simulink model "ls_fault_sw_4rt_10khz_bis"  (R2025a)
settings: Solver=VariableStepAuto  StartTime=0.0  StopTime=0.3  MaxStep=1/10e3  RelTol=1e-3
values from neighbouring files (symbols this model uses):
  Tsmpl = 1/(ovsmpl*fsw)    (= 5e-06)    [sim_ls_fault_init_4rt_10khz.m]
undefined symbols (not defined in the file or in its folder): plecs
settings Model: Creator=mem21  LastModifiedBy=mem21
settings DataIOCC: ReturnWorkspaceOutputs=off
settings OptimizationCC: DefaultParameterBehavior=Inlined  GainParamInheritBuiltInType=on  UseFloatMulNetSlope=on  InlineInvariantSignals=on  EfficientFloat2IntCast=on
settings DebuggingCC: SignalInfNanChecking=warning  AlgebraicLoopMsg=none
settings RTWCC: GenCodeOnly=on  BuildConfiguration=Faster Runs
settings GRTTargetCC: MatFileLogging=off  SupportNonFinite=off

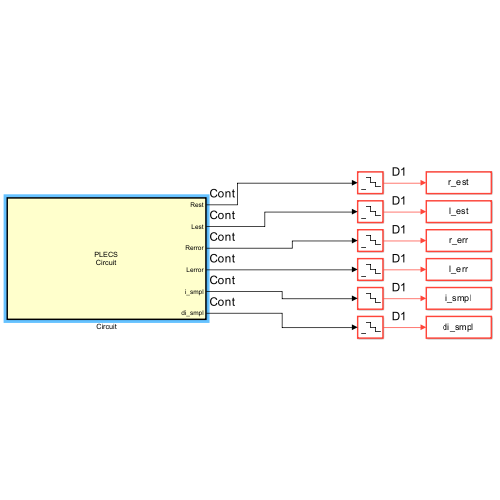
[thumbnail: Simulink's stored preview of the top-level diagram]
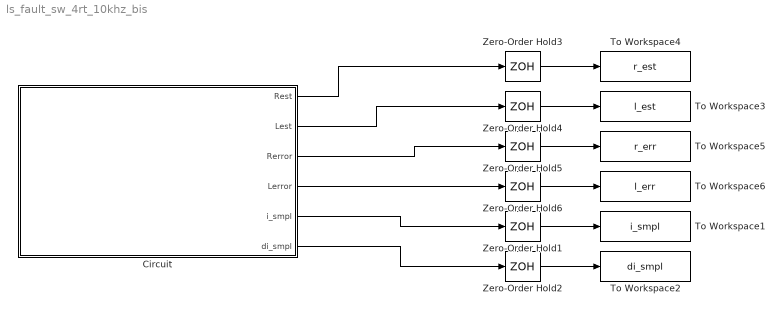
== system ls_fault_sw_4rt_10khz_bis ==
  Circuit : Subsystem  LoadFcn=plecs('sl', 200);  InitFcn=plecs('sl', 214);  StartFcn=plecs('sl', 208);  StopFcn=plecs('sl', 209);  mask(PlecsCircuit){PLECSData=<binary blob, 34132 chars, not shown>}
      mask prompts: PLECSData "PLECS Data (Do not delete or modify!)"
      mask init:
      | % PLACE CUSTOM INITIALIZATIONS ABOVE
      | % DO NOT REMOVE
      | plecs('sl', 215);
      | % DO NOT REMOVE
      settings: CopyFcn=plecs('sl', 203);  DeleteFcn=plecs('sl', 205);  UndoDeleteFcn=plecs('sl', 206);  PreSaveFcn=plecs('sl', 211);  PostSaveFcn=plecs('sl', 201);  NameChangeFcn=plecs('sl', 210);  DestroyFcn=plecs('sl', 207);  PreCopyFcn=plecs('sl', 216);  OpenFcn=plecs('sl', 202);  ErrorFcn=plerrorfcn
      mask Help: eval('plecs(''help'', ''qthelp:///creatingacircuit.html'')')
      mask Display: disp('PLECS\nCircuit')
  To Workspace1 : ToWorkspace  VariableName=i_smpl  SaveFormat=Structure With Time  SampleTime=-1
  To Workspace2 : ToWorkspace  VariableName=di_smpl  SaveFormat=Structure With Time  SampleTime=-1
  To Workspace3 : ToWorkspace  VariableName=l_est  SaveFormat=Structure With Time  SampleTime=-1
  To Workspace4 : ToWorkspace  VariableName=r_est  SaveFormat=Structure With Time  SampleTime=-1
  To Workspace5 : ToWorkspace  VariableName=r_err  SaveFormat=Structure With Time  SampleTime=-1
  To Workspace6 : ToWorkspace  VariableName=l_err  SaveFormat=Structure With Time  SampleTime=-1
  Zero-Order Hold{1..6} (6 alike) : ZeroOrderHold  SampleTime=Tsmpl
  wires:
  Zero-Order Hold4/1 -> To Workspace3/1
  Zero-Order Hold5/1 -> To Workspace5/1
  Zero-Order Hold3/1 -> To Workspace4/1
  Zero-Order Hold6/1 -> To Workspace6/1
  Circuit/1(Rest) -> Zero-Order Hold3/1
  Circuit/2(Lest) -> Zero-Order Hold4/1
  Circuit/3(Rerror) -> Zero-Order Hold5/1
  Circuit/4(Lerror) -> Zero-Order Hold6/1
  Zero-Order Hold1/1 -> To Workspace1/1
  Zero-Order Hold2/1 -> To Workspace2/1
  Circuit/5(i_smpl) -> Zero-Order Hold1/1
  Circuit/6(di_smpl) -> Zero-Order Hold2/1

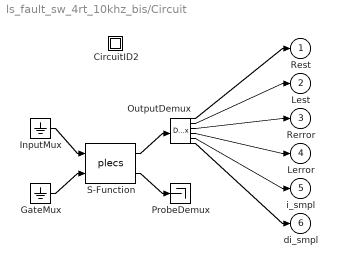
== system ls_fault_sw_4rt_10khz_bis/Circuit ==
  " CircuitID2 " : Subsystem
  " GateMux " : Ground
  " InputMux " : Ground
  " OutputDemux " : Demux  Outputs=[ 1 1 1 1 1 1 ]
  " ProbeDemux " : Terminator
  " S-Function " : S-Function  FunctionName=plecs  SFunctionDeploymentMode=off  EnableBusSupport=off
  Rest : Outport  PortDimensions=1
  Lest : Outport  Port=2  PortDimensions=1
  Rerror : Outport  Port=3  PortDimensions=1
  Lerror : Outport  Port=4  PortDimensions=1
  i_smpl : Outport  Port=5  PortDimensions=1
  di_smpl : Outport  Port=6  PortDimensions=1
  wires:
  " InputMux "/1 -> " S-Function "/1
  " GateMux "/1 -> " S-Function "/2
  " S-Function "/1 -> " OutputDemux "/1
  " S-Function "/2 -> " ProbeDemux "/1
  " OutputDemux "/1 -> Rest/1
  " OutputDemux "/2 -> Lest/1
  " OutputDemux "/3 -> Rerror/1
  " OutputDemux "/4 -> Lerror/1
  " OutputDemux "/5 -> i_smpl/1
  " OutputDemux "/6 -> di_smpl/1

== system ls_fault_sw_4rt_10khz_bis/Circuit/ CircuitID2  ==
